simulink model "run_small_function_cov"  (R2022b)
settings: Solver=FixedStepDiscrete  StartTime=0.0  StopTime=1300  RelTol=1e-3
libraries: ece1718_small_function x21, hdlsllib x1
settings Model: DataTypeOverride=Off  Creator=kevin  LastModifiedBy=kevin
settings OptimizationCC: BlockReduction=off  ConditionallyExecuteInputs=off  DefaultParameterBehavior=Inlined  InheritOutputTypeSmallerThanSingle=on
settings DebuggingCC: AlgebraicLoopMsg=error  SingleTaskRateTransMsg=error
settings HardwareCC: ProdBitPerPointer=32  ProdBitPerSizeT=32  ProdBitPerPtrDiffT=32  ProdLargestAtomicFloat=None  ProdIntDivRoundTo=Undefined  ProdEndianess=Unspecified  ProdWordSize=32  ProdHWDeviceType=ASIC/FPGA->ASIC/FPGA  TargetBitPerLong=64  TargetBitPerPointer=64  TargetBitPerSizeT=64  TargetBitPerPtrDiffT=64  TargetLongLongMode=on  TargetIntDivRoundTo=Zero  TargetEndianess=LittleEndian  TargetWordSize=64  TargetHWDeviceType=Custom Processor->MATLAB Host Computer  ProdEqTarget=off

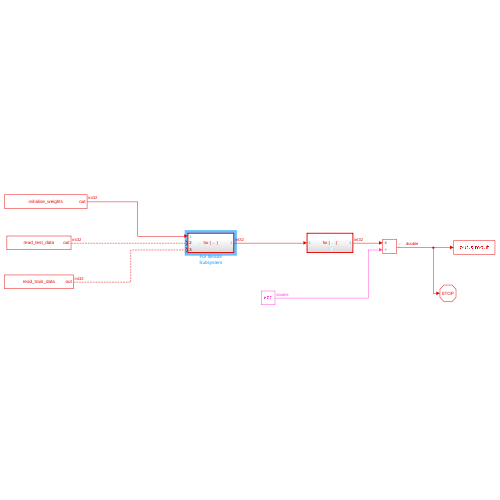
[thumbnail: Simulink's stored preview of the top-level diagram]
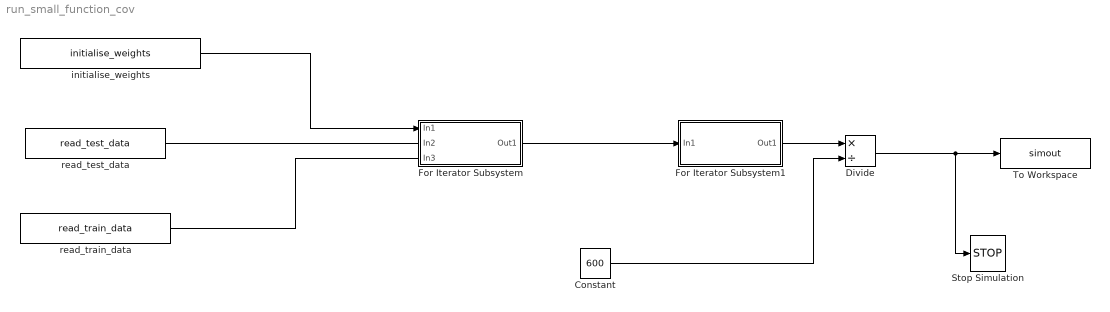
== system run_small_function_cov ==
  Constant : Constant  Value=600
  Divide : Product  Inputs=*/  OutDataTypeStr=double
  For Iterator Subsystem : Subsystem  TreatAsAtomicUnit=on
  For Iterator Subsystem1 : Subsystem  TreatAsAtomicUnit=on
  Stop Simulation : Stop
  To Workspace : ToWorkspace  VariableName=simout  SaveFormat=Timeseries  SampleTime=-1
  initialise_weights : ece1718_small_function/initialise_weights  SampleTime=-1
      settings: SourceProductName=ece1718_small_function
  read_test_data : ece1718_small_function/read_test_data  SampleTime=-1
      settings: SourceProductName=ece1718_small_function
  read_train_data : ece1718_small_function/read_train_data  SampleTime=-1
      settings: SourceProductName=ece1718_small_function
  wires:
  For Iterator Subsystem/1(Out1) -> For Iterator Subsystem1/1(In1)
  read_test_data/1 -> ?
  read_train_data/1 -> ?
  For Iterator Subsystem1/1(Out1) -> Divide/1
  Constant/1 -> Divide/2
  Divide/1 -> Stop Simulation/1, To Workspace/1
  initialise_weights/1 -> For Iterator Subsystem/1(In1)

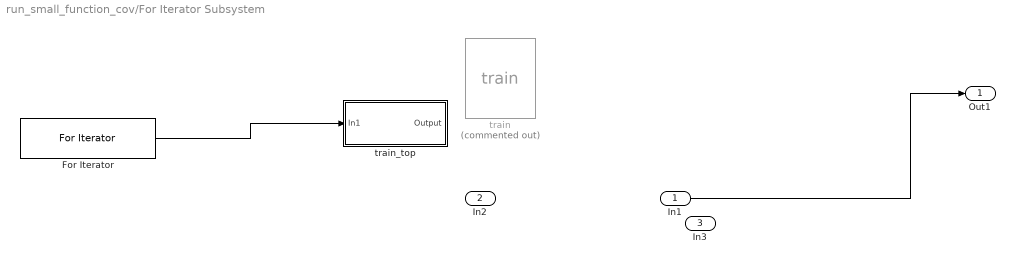
== system run_small_function_cov/For Iterator Subsystem ==
  In1 : Inport
  In2 : Inport  Port=2
  In3 : Inport  Port=3
  For Iterator : ForIterator  ResetStates=reset  IndexMode=Zero-based
  train : ece1718_small_function/train  Commented=on  SampleTime=-1
      settings: SourceProductName=ece1718_small_function
  train_top : Subsystem  TreatAsAtomicUnit=on
  Out1 : Outport
  wires:
  In1/1 -> Out1/1
  For Iterator/1 -> train_top/1(In1)

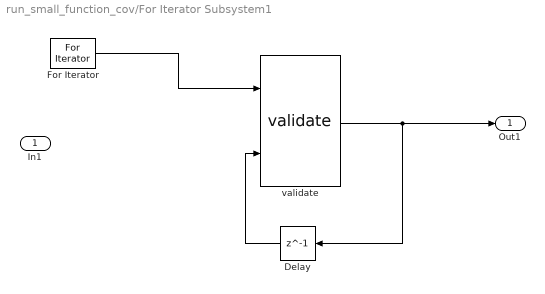
== system run_small_function_cov/For Iterator Subsystem1 ==
  In1 : Inport
  Delay : Delay  DelayLength=1  InitialCondition=0
  For Iterator : ForIterator  IterationLimit=600  IndexMode=Zero-based
  validate : ece1718_small_function/validate  SampleTime=-1
      settings: SourceProductName=ece1718_small_function
  Out1 : Outport
  wires:
  validate/1 -> Delay/1, Out1/1
  For Iterator/1 -> validate/1
  Delay/1 -> validate/2

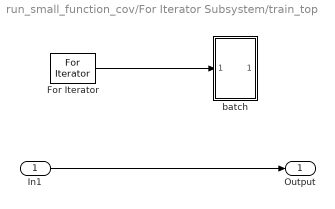
== system run_small_function_cov/For Iterator Subsystem/train_top ==
  In1 : Inport
  For Iterator : ForIterator  ResetStates=reset  IterationLimit=200  IndexMode=Zero-based
  batch : Subsystem
  Output : Outport
  wires:
  For Iterator/1 -> batch/1(Input)
  In1/1 -> Output/1

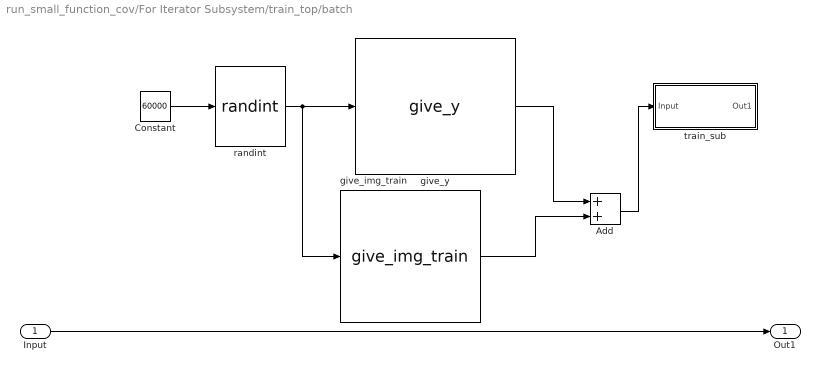
== system run_small_function_cov/For Iterator Subsystem/train_top/batch ==
  Input : Inport
  Add : Sum
  Constant : Constant  Value=60000  OutDataTypeStr=int32
  give_img_train : ece1718_small_function/give_img_train  SampleTime=-1
      settings: SourceProductName=ece1718_small_function
  give_y : ece1718_small_function/give_y  SampleTime=-1
      settings: SourceProductName=ece1718_small_function
  randint : ece1718_small_function/randint  SampleTime=-1
      settings: SourceProductName=ece1718_small_function
  train_sub : Subsystem
      settings: LibrarySourceBlock=|
      | hdlsllib/Ports &
      | Subsystems/Subsystem
  Out1 : Outport
  wires:
  give_y/1 -> Add/1
  randint/1 -> give_img_train/1, give_y/1
  Constant/1 -> randint/1
  Input/1 -> Out1/1
  give_img_train/1 -> Add/2
  Add/1 -> train_sub/1(Input)

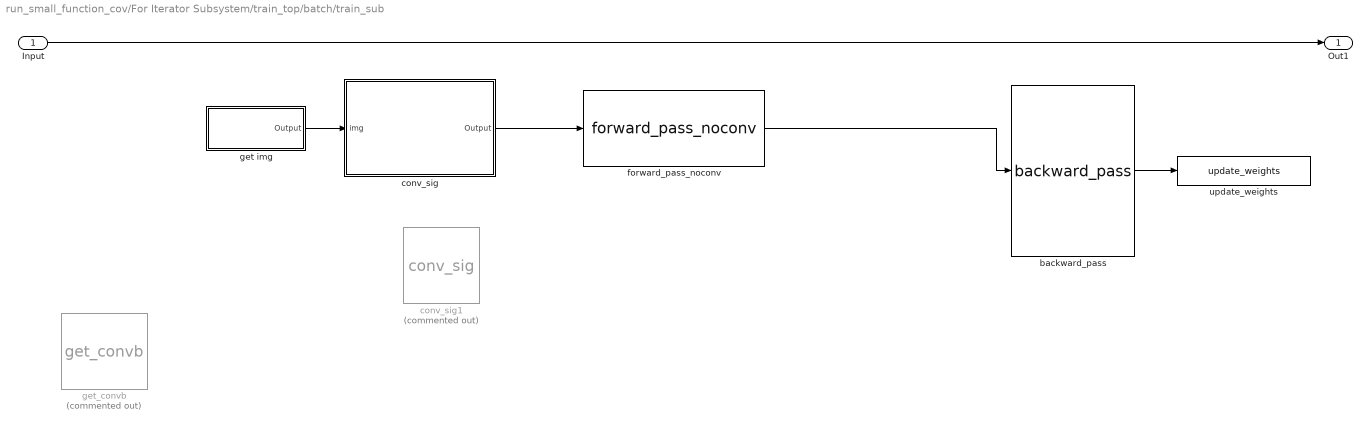
== system run_small_function_cov/For Iterator Subsystem/train_top/batch/train_sub ==
  Input : Inport
  backward_pass : ece1718_small_function/backward_pass  SampleTime=-1
      settings: SourceProductName=ece1718_small_function
  conv_sig : Subsystem
      settings: LibrarySourceBlock=|
      | hdlsllib/Ports &
      | Subsystems/Subsystem
  conv_sig1 : ece1718_small_function/conv_sig  Commented=on  SampleTime=-1
      settings: SourceProductName=ece1718_small_function
  forward_pass_noconv : ece1718_small_function/forward_pass_noconv  SampleTime=-1
      settings: SourceProductName=ece1718_small_function
  get img : Subsystem  TreatAsAtomicUnit=on
  get_convb : ece1718_small_function/get_convb  Commented=on  SampleTime=-1
      settings: SourceProductName=ece1718_small_function
  update_weights : ece1718_small_function/update_weights  SampleTime=-1
      settings: SourceProductName=ece1718_small_function
  Out1 : Outport
  wires:
  forward_pass_noconv/1 -> backward_pass/1
  backward_pass/1 -> update_weights/1
  Input/1 -> Out1/1
  get img/1(Output) -> conv_sig/1(img)
  conv_sig/1(Output) -> forward_pass_noconv/1

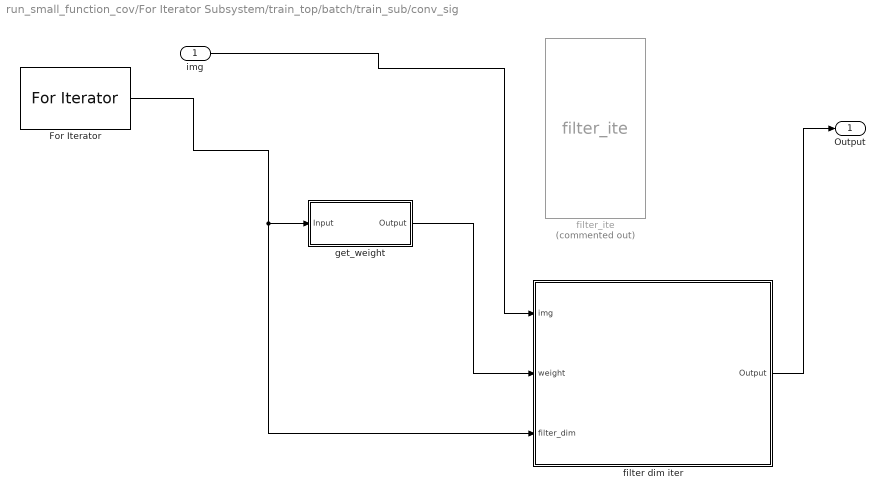
== system run_small_function_cov/For Iterator Subsystem/train_top/batch/train_sub/conv_sig ==
  img : Inport
  For Iterator : ForIterator  ResetStates=reset  IndexMode=Zero-based
  "filter dim iter " : Subsystem  TreatAsAtomicUnit=on
  filter_ite : ece1718_small_function/filter_ite  Commented=on  SampleTime=-1
      settings: SourceProductName=ece1718_small_function
  "get_weight " : Subsystem  TreatAsAtomicUnit=on
  Output : Outport
  wires:
  For Iterator/1 -> "filter dim iter "/3(filter_dim), "get_weight "/1(Input)
  img/1 -> "filter dim iter "/1(img)
  "filter dim iter "/1(Output) -> Output/1
  "get_weight "/1(Output) -> "filter dim iter "/2(weight)

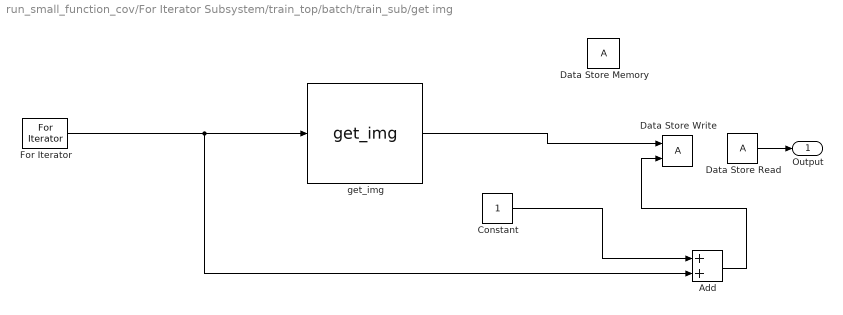
== system run_small_function_cov/For Iterator Subsystem/train_top/batch/train_sub/get img ==
  Add : Sum  OutDataTypeStr=int32
  Constant : Constant  OutDataTypeStr=int32
  Data Store Memory : DataStoreMemory  WriteAfterWriteMsg=warning  ShowAdditionalParam=off  OutDataTypeStr=uint8  Dimensions=1120
  Data Store Read : DataStoreRead  IndexOptions=Index vector (dialog)  Indices=1  OutputSizes=1
  Data Store Write : DataStoreWrite  EnableIndexing=on  IndexOptions=Index vector (port)  Indices=1  OutputSizes=1
  For Iterator : ForIterator  ResetStates=reset  IterationLimit=1120  IndexMode=Zero-based
  get_img : ece1718_small_function/get_img  SampleTime=-1
      settings: SourceProductName=ece1718_small_function
  Output : Outport
  wires:
  For Iterator/1 -> Add/2, get_img/1
  get_img/1 -> Data Store Write/1
  Data Store Read/1 -> Output/1
  Constant/1 -> Add/1
  Add/1 -> Data Store Write/2

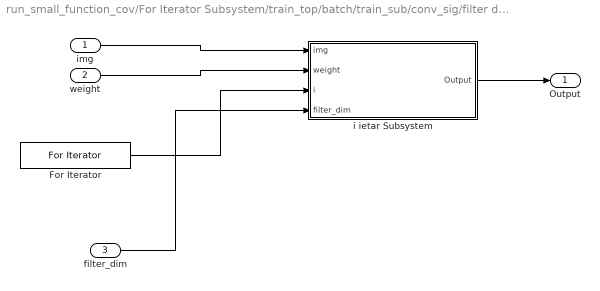
== system run_small_function_cov/For Iterator Subsystem/train_top/batch/train_sub/conv_sig/filter dim iter  ==
  img : Inport
  weight : Inport  Port=2
  filter_dim : Inport  Port=3
  For Iterator : ForIterator  ResetStates=reset  IterationLimit=28  IndexMode=Zero-based
  i ietar Subsystem : Subsystem  TreatAsAtomicUnit=on
  Output : Outport
  wires:
  img/1 -> i ietar Subsystem/1(img)
  weight/1 -> i ietar Subsystem/2(weight)
  For Iterator/1 -> i ietar Subsystem/3(i)
  filter_dim/1 -> i ietar Subsystem/4(filter_dim)
  i ietar Subsystem/1(Output) -> Output/1

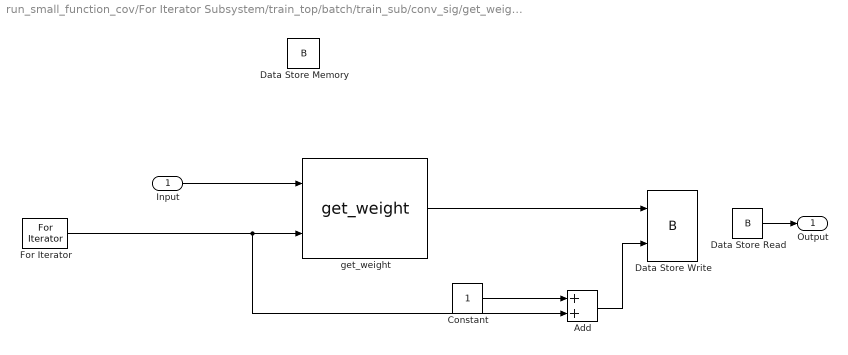
== system run_small_function_cov/For Iterator Subsystem/train_top/batch/train_sub/conv_sig/get_weight  ==
  Input : Inport
  Add : Sum  OutDataTypeStr=int32
  Constant : Constant  OutDataTypeStr=int32
  Data Store Memory : DataStoreMemory  DataStoreName=B  ReadBeforeWriteMsg=warning  WriteAfterWriteMsg=warning  ShowAdditionalParam=off  OutDataTypeStr=double  Dimensions=49
  Data Store Read : DataStoreRead  DataStoreName=B  IndexOptions=Index vector (dialog)  Indices=1  OutputSizes=1
  Data Store Write : DataStoreWrite  DataStoreName=B  DataStoreElements=B  EnableIndexing=on  IndexOptions=Index vector (port)  Indices=1  OutputSizes=1
  For Iterator : ForIterator  ResetStates=reset  IterationLimit=49  IndexMode=Zero-based
  get_weight : ece1718_small_function/get_weight  SampleTime=-1
      settings: SourceProductName=ece1718_small_function
  Output : Outport
  wires:
  For Iterator/1 -> Add/2, get_weight/2
  Input/1 -> get_weight/1
  Data Store Read/1 -> Output/1
  Constant/1 -> Add/1
  Add/1 -> Data Store Write/2
  get_weight/1 -> Data Store Write/1

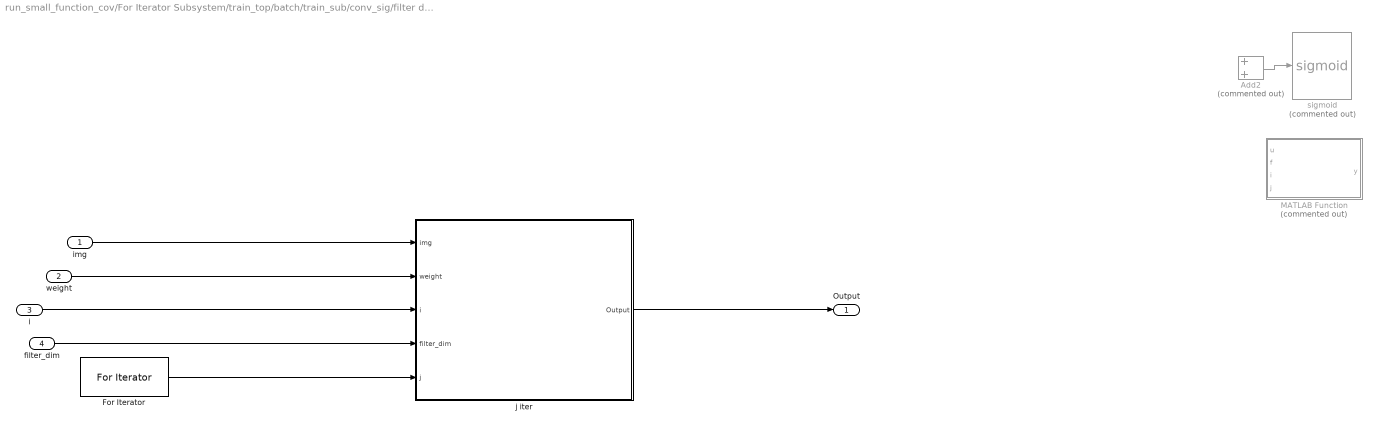
== system run_small_function_cov/For Iterator Subsystem/train_top/batch/train_sub/conv_sig/filter dim iter /i ietar Subsystem ==
  img : Inport
  weight : Inport  Port=2
  i : Inport  Port=3
  filter_dim : Inport  Port=4
  Add2 : Sum  Commented=on
  For Iterator : ForIterator  ResetStates=reset  IterationLimit=28  IndexMode=Zero-based
  MATLAB Function : MATLAB Function  Commented=on  TreatAsAtomicUnit=on
  j iter : Subsystem
  sigmoid : ece1718_small_function/sigmoid  Commented=on  SampleTime=-1
      settings: SourceProductName=ece1718_small_function
  Output : Outport
  wires:
  Add2/1 -> sigmoid/1
  For Iterator/1 -> j iter/5(j)
  filter_dim/1 -> j iter/4(filter_dim)
  i/1 -> j iter/3(i)
  weight/1 -> j iter/2(weight)
  img/1 -> j iter/1(img)
  j iter/1(Output) -> Output/1

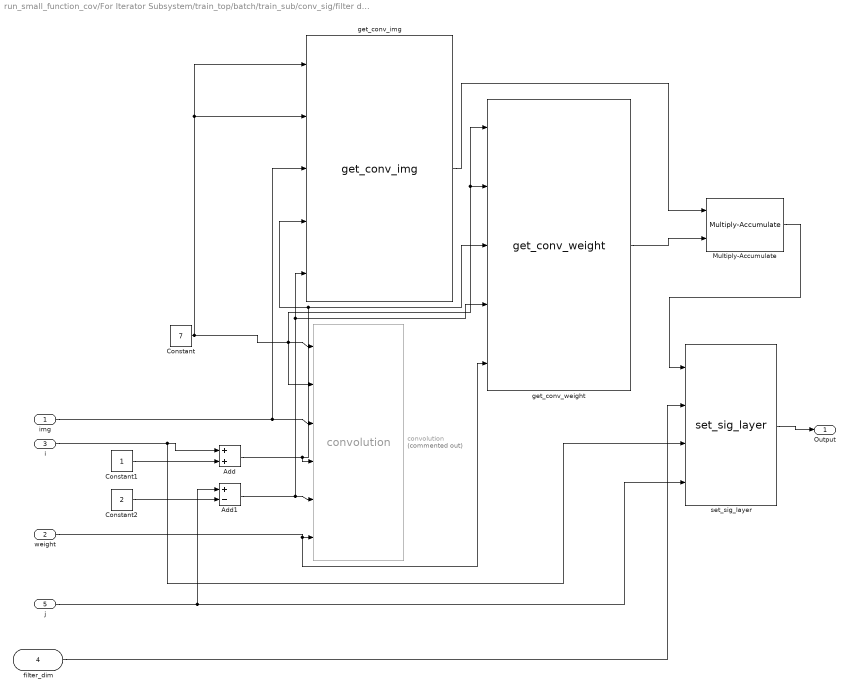
== system run_small_function_cov/For Iterator Subsystem/train_top/batch/train_sub/conv_sig/filter dim iter /i ietar Subsystem/j iter ==
  img : Inport
  weight : Inport  Port=2
  i : Inport  Port=3
  filter_dim : Inport  Port=4
  j : Inport  Port=5
  Add : Sum  OutDataTypeStr=int32
  Add1 : Sum  Inputs=+-  OutDataTypeStr=int32
  Constant : Constant  Value=7  OutDataTypeStr=int32
  Constant1 : Constant  OutDataTypeStr=int32
  Constant2 : Constant  Value=2  OutDataTypeStr=int32
  Multiply-Accumulate : hdlsllib/HDL Operations/Multiply-Accumulate  opMode=Vector  initValueSetting=Dialog  initValue=0  initValueSetting2=Dialog  initValue2=0  initValueSetting3=Dialog  initValue3=0  num_samples=2  RndMeth2=Floor  RndMeth3=Floor  datatype2=Inherit: Inherit via back propagation  datatype3=Inherit: Inherit via back propagation  validOut=on  endInandOut=on  startOut=on  countOut=on  dim=-1  DoSatur=off  parallel=off
  convolution : ece1718_small_function/convolution  Commented=on  SampleTime=-1
      settings: SourceProductName=ece1718_small_function
  get_conv_img : ece1718_small_function/get_conv_img  SampleTime=-1
      settings: SourceProductName=ece1718_small_function
  get_conv_weight : ece1718_small_function/get_conv_weight  SampleTime=-1
      settings: SourceProductName=ece1718_small_function
  set_sig_layer : ece1718_small_function/set_sig_layer  SampleTime=-1
      settings: SourceProductName=ece1718_small_function
  Output : Outport
  wires:
  Constant2/1 -> Add1/2
  img/1 -> convolution/3, get_conv_img/3
  Constant1/1 -> Add/2
  Add1/1 -> get_conv_img/5, get_conv_weight/4, convolution/5
  Add/1 -> get_conv_img/4, get_conv_weight/3, convolution/4
  i/1 -> set_sig_layer/3, Add/1
  filter_dim/1 -> set_sig_layer/2
  Constant/1 -> get_conv_weight/1, get_conv_weight/2, convolution/2, convolution/1, get_conv_img/1, get_conv_img/2
  weight/1 -> get_conv_weight/5, convolution/6
  j/1 -> Add1/1, set_sig_layer/4
  set_sig_layer/1 -> Output/1
  get_conv_img/1 -> Multiply-Accumulate/1
  get_conv_weight/1 -> Multiply-Accumulate/2
  Multiply-Accumulate/1 -> set_sig_layer/1

== matlab function run_small_function_cov/For Iterator Subsystem/train_top/batch/train_sub/conv_sig/filter dim iter /i ietar Subsystem/MATLAB Function ==
  data: u input; y output; f input; i input; j input
function y = fcn(u,f,i,j)

y = u(f+1,i+1,j+1);
end
